simulink model "step5"  (R2021b)
settings: Solver=VariableStepAuto  StartTime=0.0  StopTime=10.0  RelTol=1e-3
settings Model: Creator=just cookie file  LastModifiedBy=just cookie file

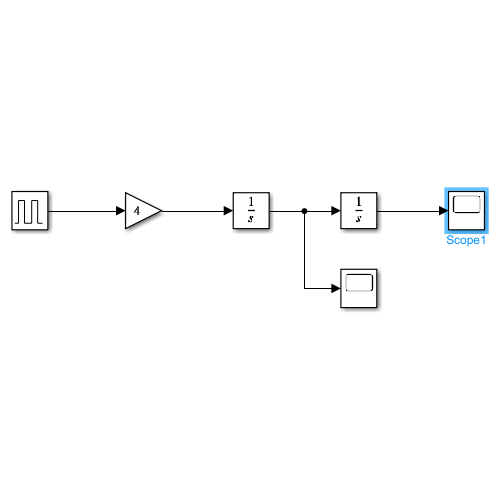
[thumbnail: Simulink's stored preview of the top-level diagram]
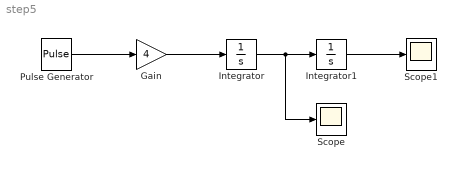
== system step5 ==
  Gain : Gain  Gain=4
  Integrator : Integrator
  Integrator1 : Integrator
  Pulse Generator : DiscretePulseGenerator  PulseType=Time based  Period=0.5  PulseWidth=0.1
  Scope : Scope
  Scope1 : Scope
  wires:
  Pulse Generator/1 -> Gain/1
  Gain/1 -> Integrator/1
  Integrator/1 -> Scope/1, Integrator1/1
  Integrator1/1 -> Scope1/1
